simulink model "diff_drive_sim"  (R2021b)
settings: Solver=FixedStepAuto  StartTime=0.0  StopTime=489.5  FixedStep=0.1  RelTol=1e-3
undefined symbols (not defined in the file): a, theta0, w, x0, y0
settings Model: Creator=olivier  LastModifiedBy=sakth
settings SolverCC: ZeroCrossAlgorithm=Adaptive  AlgebraicLoopSolver=TrustRegion
settings DataIOCC: ReturnWorkspaceOutputs=off
settings DebuggingCC: MaskedZcDiagnostic=none  SFMachineParentedDataDiag=warning  ArithmeticOperatorsInVariantConditions=warning
settings SFSimCC: CustomCodeUndefinedFunction=UseInterfaceOnly

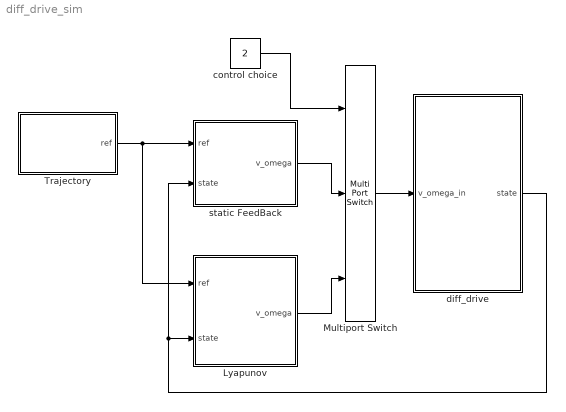
== system diff_drive_sim ==
  Lyapunov : Subsystem
  Multiport Switch : MultiPortSwitch  Inputs=2
  Trajectory : Subsystem  TreatAsAtomicUnit=on
  control choice : Constant  Value=2
  diff_drive : Subsystem  mask{base=0.5, base_error=0, radius=0.2, radius_error=0, omega_max=80}
      mask prompts: base_error "Base error in percent"; radius_error "Radius error in percent"; omega_max "Wheel Max Velocity"
  static FeedBack : Subsystem
  wires:
  Trajectory/1(ref) -> Lyapunov/1(ref), static FeedBack/1(ref)
  static FeedBack/1(v_omega) -> Multiport Switch/2
  Multiport Switch/1 -> diff_drive/1(v_omega_in)
  control choice/1 -> Multiport Switch/1
  diff_drive/1(state) -> Lyapunov/2(state), static FeedBack/2(state)
  Lyapunov/1(v_omega) -> Multiport Switch/3

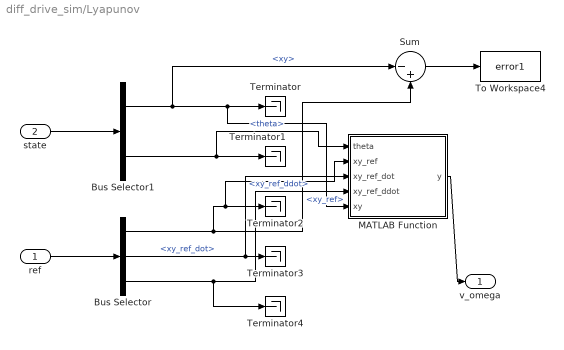
== system diff_drive_sim/Lyapunov ==
  ref : Inport
  state : Inport  Port=2
  Bus Selector : BusSelector  OutputSignals=xy_ref,xy_ref_dot,xy_ref_ddot
  Bus Selector1 : BusSelector  OutputSignals=xy,theta
  MATLAB Function : MATLAB Function  TreatAsAtomicUnit=on
  Sum : Sum  Inputs=|-+
  Terminator{,1..4} (5 alike) : Terminator
  To Workspace4 : ToWorkspace  VariableName=error1  SampleTime=-1
      settings: Save2DSignal=2-D array (concatenate along first dimension)
  v_omega : Outport  VectorParamsAs1DForOutWhenUnconnected=off
  wires:
  ref/1 -> Bus Selector/1
  state/1 -> Bus Selector1/1
  Bus Selector/2 -> MATLAB Function/3(xy_ref_dot), Terminator3/1  "<xy_ref_dot>"
  Bus Selector/1 -> Sum/2, MATLAB Function/2(xy_ref), Terminator2/1  "<xy_ref>"
  Bus Selector/3 -> MATLAB Function/4(xy_ref_ddot), Terminator4/1  "<xy_ref_ddot>"
  Bus Selector1/1 -> Sum/1, MATLAB Function/5(xy), Terminator/1  "<xy>"
  Bus Selector1/2 -> MATLAB Function/1(theta), Terminator1/1  "<theta>"
  MATLAB Function/1(y) -> v_omega/1
  Sum/1 -> To Workspace4/1

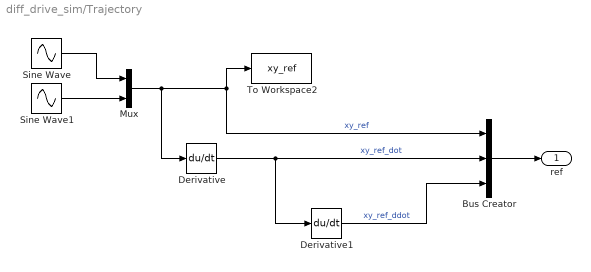
== system diff_drive_sim/Trajectory ==
  Bus Creator : BusCreator  Inputs=3
  Derivative : Derivative
  Derivative1 : Derivative
  Mux : Mux  Inputs=2
  Sine Wave : Sin  Amplitude=a  Frequency=w  Phase=pi/2  SampleTime=0
  Sine Wave1 : Sin  Amplitude=a  Frequency=w  SampleTime=0
  To Workspace2 : ToWorkspace  VariableName=xy_ref  SampleTime=-1
      settings: Save2DSignal=2-D array (concatenate along first dimension)
  ref : Outport  VectorParamsAs1DForOutWhenUnconnected=off
  wires:
  Bus Creator/1 -> ref/1
  Mux/1 -> Derivative/1, Bus Creator/1, To Workspace2/1  "xy_ref"
  Derivative/1 -> Bus Creator/2, Derivative1/1  "xy_ref_dot"
  Derivative1/1 -> Bus Creator/3  "xy_ref_ddot"
  Sine Wave1/1 -> Mux/2
  Sine Wave/1 -> Mux/1

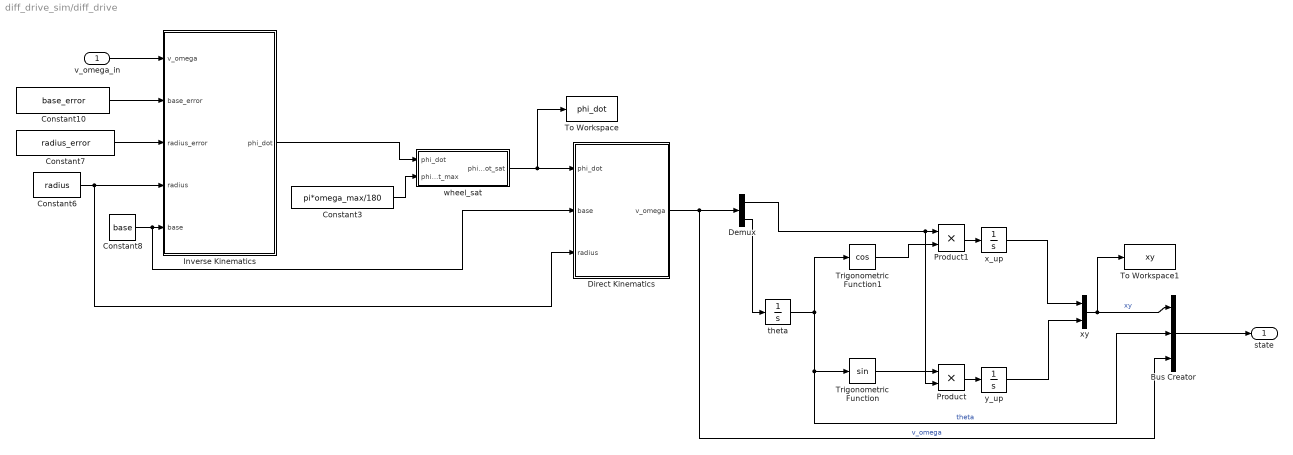
== system diff_drive_sim/diff_drive ==
  v_omega_in : Inport
  Bus Creator : BusCreator  Inputs=3
  Constant10 : Constant  Value=base_error
  Constant3 : Constant  Value=pi*omega_max/180
  Constant6 : Constant  Value=radius
  Constant7 : Constant  Value=radius_error
  Constant8 : Constant  Value=base
  Demux : Demux  Outputs=2
  Direct Kinematics : MATLAB Function  TreatAsAtomicUnit=on
  Inverse Kinematics : MATLAB Function  TreatAsAtomicUnit=on
  Product : Product
  Product1 : Product
  To Workspace : ToWorkspace  VariableName=phi_dot  SampleTime=-1
      settings: Save2DSignal=2-D array (concatenate along first dimension)
  To Workspace1 : ToWorkspace  VariableName=xy  SampleTime=-1
      settings: Save2DSignal=2-D array (concatenate along first dimension)
  Trigonometric Function : Trigonometry
  Trigonometric Function1 : Trigonometry  Operator=cos
  theta : Integrator  InitialCondition=theta0
  wheel_sat : Subsystem
  x_up : Integrator  InitialCondition=x0
  xy : Mux  Inputs=2
  y_up : Integrator  InitialCondition=y0
  state : Outport  VectorParamsAs1DForOutWhenUnconnected=off
  wires:
  theta/1 -> Trigonometric Function1/1, Trigonometric Function/1, Bus Creator/2  "theta"
  Trigonometric Function1/1 -> Product1/2
  Trigonometric Function/1 -> Product/1
  Product/1 -> y_up/1
  Product1/1 -> x_up/1
  x_up/1 -> xy/1
  Constant3/1 -> wheel_sat/2(phi_dot_max)
  Direct Kinematics/1(v_omega) -> Bus Creator/3, Demux/1  "v_omega"
  Demux/1 -> Product/2, Product1/1
  Demux/2 -> theta/1
  y_up/1 -> xy/2
  wheel_sat/1(phi_dot_sat) -> Direct Kinematics/1(phi_dot), To Workspace/1
  xy/1 -> Bus Creator/1, To Workspace1/1  "xy"
  Bus Creator/1 -> state/1
  Inverse Kinematics/1(phi_dot) -> wheel_sat/1(phi_dot)
  v_omega_in/1 -> Inverse Kinematics/1(v_omega)
  Constant10/1 -> Inverse Kinematics/2(base_error)
  Constant7/1 -> Inverse Kinematics/3(radius_error)
  Constant6/1 -> Inverse Kinematics/4(radius), Direct Kinematics/3(radius)
  Constant8/1 -> Direct Kinematics/2(base), Inverse Kinematics/5(base)

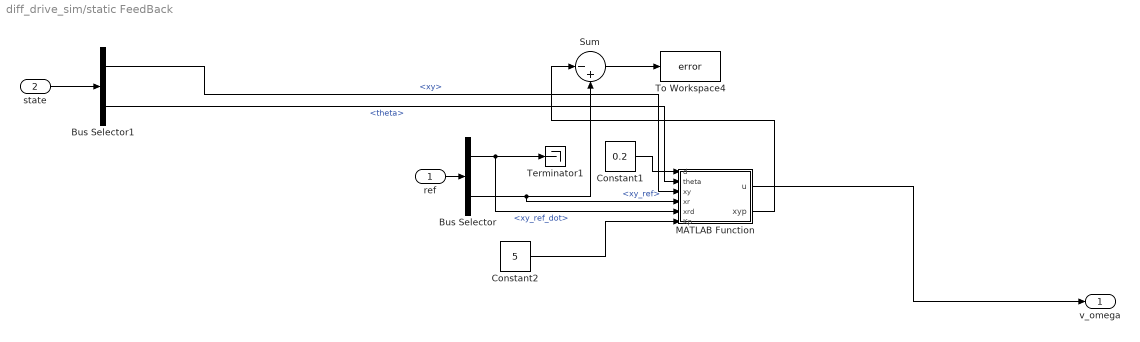
== system diff_drive_sim/static FeedBack ==
  ref : Inport
  state : Inport  Port=2
  Bus Selector : BusSelector  OutputSignals=xy_ref_dot,xy_ref
  Bus Selector1 : BusSelector  OutputSignals=xy,theta
  Constant1 : Constant  Value=0.2
  Constant2 : Constant  Value=5
  MATLAB Function : MATLAB Function  TreatAsAtomicUnit=on
  Sum : Sum  Inputs=|-+
  Terminator1 : Terminator
  To Workspace4 : ToWorkspace  VariableName=error  SampleTime=-1
      settings: Save2DSignal=2-D array (concatenate along first dimension)
  v_omega : Outport  VectorParamsAs1DForOutWhenUnconnected=off
  wires:
  ref/1 -> Bus Selector/1
  state/1 -> Bus Selector1/1
  Bus Selector/2 -> MATLAB Function/4(xr), Sum/2  "<xy_ref>"
  Bus Selector1/1 -> MATLAB Function/3(xy)  "<xy>"
  Sum/1 -> To Workspace4/1
  MATLAB Function/1(u) -> v_omega/1
  Bus Selector1/2 -> MATLAB Function/2(theta)  "<theta>"
  Bus Selector/1 -> MATLAB Function/5(xrd), Terminator1/1  "<xy_ref_dot>"
  Constant1/1 -> MATLAB Function/1(d)
  Constant2/1 -> MATLAB Function/6(Kp)
  MATLAB Function/2(xyp) -> Sum/1

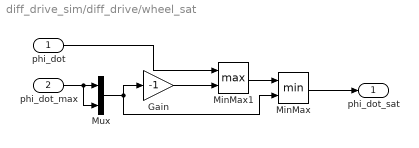
== system diff_drive_sim/diff_drive/wheel_sat ==
  phi_dot : Inport
  phi_dot_max : Inport  Port=2
  Gain : Gain  Gain=-1
  MinMax : MinMax  Inputs=2
  MinMax1 : MinMax  Function=max  Inputs=2
  Mux : Mux  Inputs=2
  phi_dot_sat : Outport  VectorParamsAs1DForOutWhenUnconnected=off
  wires:
  Gain/1 -> MinMax1/2
  MinMax/1 -> phi_dot_sat/1
  phi_dot_max/1 -> Mux/2, Mux/1
  phi_dot/1 -> MinMax1/1
  MinMax1/1 -> MinMax/1
  Mux/1 -> MinMax/2, Gain/1

== matlab function diff_drive_sim/diff_drive/Inverse Kinematics ==
  data: v_omega input; base_error input; radius_error input; radius input; phi_dot output; base input
function phi_dot = ik(v_omega, base_error, radius_error, radius, base)

base = base * (1+base_error*0.01);
radius = radius * (1+radius_error*0.01);

phi_dot = [(v_omega(1)+base*v_omega(2))/radius; (v_omega(1)-base*v_omega(2))/radius];

== matlab function diff_drive_sim/static FeedBack/MATLAB Function ==
  data: d input; u output; theta input; xy input; xr input; xrd input; Kp input; xyp output
function [u,xyp]  = fcn(d,theta,xy,xr,xrd,Kp)
%#codegen
xp = xy(1) + d*cos(theta)
yp = xy(2) + d*sin(theta)
xyp = [xp,yp]
K = [cos(theta) -d*sin(theta);sin(theta) d*cos(theta)]
u = inv(K)*(xrd + Kp*(xr - xy))

== matlab function diff_drive_sim/Lyapunov/MATLAB Function ==
  data: theta input; y output; xy_ref input; xy_ref_dot input; xy_ref_ddot input; xy input
function y = fcn(theta,xy_ref,xy_ref_dot,xy_ref_ddot,xy)
kx = 0.099
ky = 0.09
ktheta = 0.09

xe = cos(theta)*(xy_ref(1)-xy(1))+sin(theta)*(xy_ref(2)-xy(2))
ye = -sin(theta)*(xy_ref(1)-xy(1))+cos(theta)*(xy_ref(2)-xy(2))
thetae = wrapToPi(atan2(xy_ref(2),xy_ref(1))-theta) 


vr = xy_ref_dot(1)*cos(theta)+xy_ref_dot(2)*sin(theta)
wr = (xy_ref_dot(1)*xy_ref_ddot(2)-xy_ref_ddot(1)*xy_ref_dot(2))/(vr^2)

v = vr*cos(thetae) + kx*xe
w = wr+ky*ye*vr*sin(thetae)/thetae+ktheta*thetae

y = [v;w];

== matlab function diff_drive_sim/diff_drive/Direct Kinematics ==
  data: phi_dot input; v_omega output; base input; radius input
function v_omega = dk(phi_dot, base, radius)

v_omega = [radius*(phi_dot(1)+phi_dot(2))/2; radius*(phi_dot(1)-phi_dot(2))/(2*base)];
